simulink model "setconfig_example"  (R2017b)
settings: Solver=VariableStepAuto  StartTime=0.0  StopTime=20  RelTol=1e-3
libraries: simulink x1, smartLib x1
settings Model: Creator=tmkhoyan  LastModifiedBy=tmkhoyan

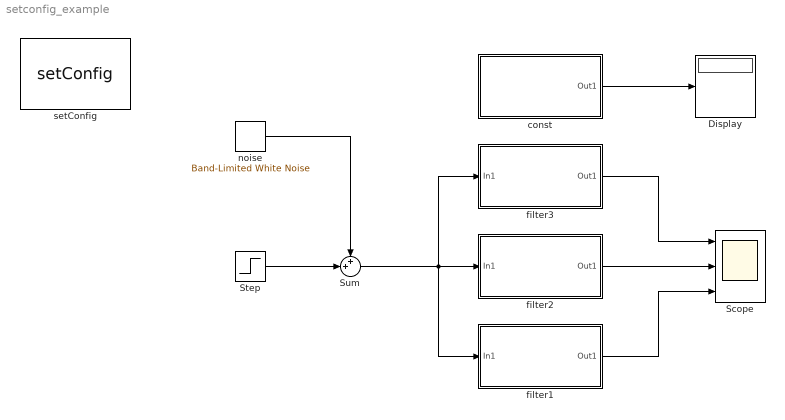
== system setconfig_example ==
  Display : Display
  Scope : Scope  NumInputPorts=3
  Step : Step  SampleTime=0
  Sum : Sum  Inputs=++|
  const : Subsystem  mask{c1=0.01, c2=0.045, c3=0.02}
      mask prompts: c1 "constant 1"; c2 "constant 2"; c3 "constant 3"
  filter1 : Subsystem
  filter2 : Subsystem
  filter3 : Subsystem
  noise : simulink/Sources/Band-Limited White Noise  Cov=0.0010  Ts=0.0012  seed=[23341]
  setConfig : smartLib/setConfig  filename='config/config.txt'
      settings: SourceProductName=smartLib
  wires:
  Sum/1 -> filter1/1(In1), filter2/1(In1), filter3/1(In1)
  filter2/1(Out1) -> Scope/2
  filter3/1(Out1) -> Scope/1
  filter1/1(Out1) -> Scope/3
  Step/1 -> Sum/2
  noise/1 -> Sum/1
  const/1(Out1) -> Display/1

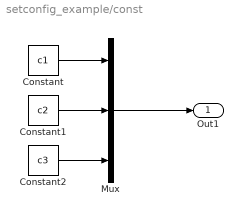
== system setconfig_example/const ==
  Constant : Constant  Value=c1
  Constant1 : Constant  Value=c2
  Constant2 : Constant  Value=c3
  Mux : Mux  Inputs=3
  Out1 : Outport
  wires:
  Constant/1 -> Mux/1
  Constant1/1 -> Mux/2
  Constant2/1 -> Mux/3
  Mux/1 -> Out1/1

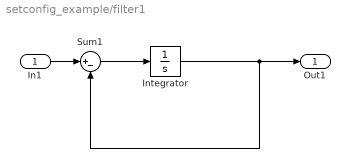
== system setconfig_example/filter1 ==
  In1 : Inport
  Integrator : Integrator  InitialCondition=2
  Sum1 : Sum  Inputs=|+-
  Out1 : Outport
  wires:
  Sum1/1 -> Integrator/1
  Integrator/1 -> Out1/1, Sum1/2
  In1/1 -> Sum1/1

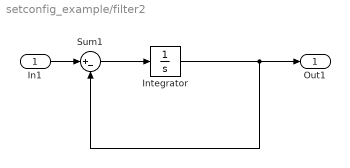
== system setconfig_example/filter2 ==
  In1 : Inport
  Integrator : Integrator  InitialCondition=-2  UpperSaturationLimit=120
  Sum1 : Sum  Inputs=|+-
  Out1 : Outport
  wires:
  In1/1 -> Sum1/1
  Integrator/1 -> Sum1/2, Out1/1
  Sum1/1 -> Integrator/1

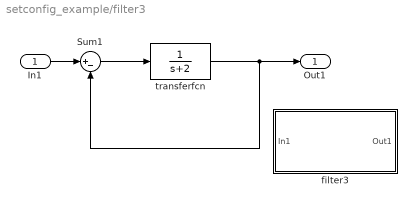
== system setconfig_example/filter3 ==
  In1 : Inport
  Sum1 : Sum  Inputs=|+-
  filter3 : Subsystem
  transferfcn : TransferFcn  Denominator=[1 2]
  Out1 : Outport
  wires:
  Sum1/1 -> transferfcn/1
  transferfcn/1 -> Out1/1, Sum1/2
  In1/1 -> Sum1/1

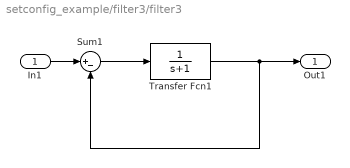
== system setconfig_example/filter3/filter3 ==
  In1 : Inport
  Sum1 : Sum  Inputs=|+-
  Transfer Fcn1 : TransferFcn  Denominator=[1 1]
  Out1 : Outport
  wires:
  Sum1/1 -> Transfer Fcn1/1
  Transfer Fcn1/1 -> Out1/1, Sum1/2
  In1/1 -> Sum1/1
